simulink model "aircraft_simulation_slc_ff"  (R2016b)
settings: Solver=ode5  StartTime=0.0  StopTime=10000  FixedStep=0.1  RelTol=1e-3  EnableMultiTasking=on
values from neighbouring files (symbols this model uses):
  chi_c = 180/pi*uu(28)    [PlotStateVariables.m]    (also in SLCWithFeedForwardAutopilot.m = uu(19,1); SLCWithFeedForwardAutopilotOLD.m = uu(21,1); SimpleCircleFollow.m = chi_0 + circle_gain_struct.flag*atan(circle_gain_struct.gain; SimpleSLCAutopilot.m = uu(17,1))
  chi_dot_c = uu(18,1)    [SLCWithFeedForwardAutopilot.m]    (also in SLCWithFeedForwardAutopilotOLD.m = control_gain_struct.Kff_course_rate*chi_dot_ff + control_gai; SimpleCircleFollow.m = scale_factor*circle_gain_struct.speed/circle_gain_struct.rad)
  h_c = uu(22)    [PlotStateVariables.m]    (also in SLCWithFeedForwardAutopilot.m = uu(17,1); SLCWithFeedForwardAutopilotOLD.m = uu(19,1); SimpleCircleFollow.m = -circle_gain_struct.center(3,1); SimpleSLCAutopilot.m = uu(18,1))
  h_dot_c = uu(16,1)    [SLCWithFeedForwardAutopilot.m]    (also in SLCWithFeedForwardAutopilotOLD.m = uu(20,1); SimpleCircleFollow.m = 0)
  Va_c = uu(23)    [PlotStateVariables.m]    (also in SLCWithFeedForwardAutopilot.m = uu(20,1); SLCWithFeedForwardAutopilotOLD.m = uu(23,1); SimpleCircleFollow.m = circle_gain_struct.speed; SimpleSLCAutopilot.m = uu(16,1))
  wind_inertial = uu(17:19, 1)    [PlotStateVariables.m]    (also in SLCWithFeedForwardAutopilot.m = uu(13:15,1); S_AircraftForcesAndMoments.m = u(17:19,1); SimpleSLCAutopilot.m = uu(13:15,1))
undefined symbols (not defined in the file or in its folder): aircraft_parameters, circle_gain_struct, control_gain_struct, DRAW_FLAG, drawAircraft, PlotStateVariables, pts, S_AircraftForcesAndMoments, SimpleCircleFollow, SLCWithFeedForwardAutopilot
libraries: aerolibobsolete x1, aerolibatmos2 x1
settings Model: Creator=beard  LastModifiedBy=ericfrew
settings DataIOCC: LimitDataPoints=on  SaveFormat=Array  SignalLoggingSaveFormat=ModelDataLogs
settings OptimizationCC: ExpressionDepthLimit=2147483647  InitFltsAndDblsToZero=on  LifeSpan=inf
settings DebuggingCC: UnderspecifiedInitializationDetection=Classic  MergeDetectMultiDrivingBlocksExec=none  SolverPrmCheckMsg=warning  FcnCallInpInsideContextMsg=warning  StateNameClashWarn=warning  SFUnexpectedBacktrackingDiag=warning  SFNoUnconditionalDefaultTransitionDiag=warning  SFExecutionAtInitializationDiag=none
settings HardwareCC: ProdBitPerPointer=32  ProdBitPerSizeT=32  ProdBitPerPtrDiffT=32  ProdLargestAtomicFloat=None  ProdIntDivRoundTo=Undefined  ProdEndianess=Unspecified  ProdWordSize=32  ProdHWDeviceType=32-bit Generic
settings ModelReferenceCC: PropagateSignalLabelsOutOfModel=off
settings GRTTargetCC: TargetLangStandard=C89/C90 (ANSI)  GeneratePreprocessorConditionals=Disable all  CombineOutputUpdateFcns=off  GRTInterface=on
settings ConfigComp: CovMetricSettings=dw  CovHtmlReporting=on  CovSaveCumulativeToWorkspaceVar=on  CovSaveSingleToWorkspaceVar=on  CovExternalEMLEnable=off  CovSFcnEnable=off

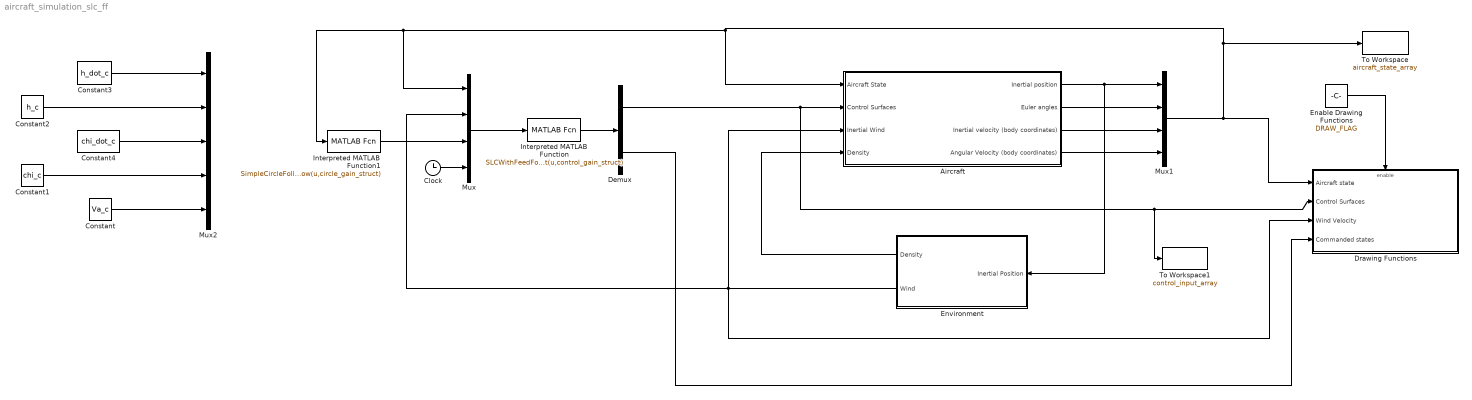
== system aircraft_simulation_slc_ff ==
  Aircraft : Subsystem
  Clock : Clock
  Constant : Constant  Value=Va_c
  Constant1 : Constant  Value=chi_c
  Constant2 : Constant  Value=h_c
  Constant3 : Constant  Value=h_dot_c
  Constant4 : Constant  Value=chi_dot_c
  Demux : Demux  Outputs=[4; 12]
  Drawing Functions : Subsystem  TreatAsAtomicUnit=on
  Enable Drawing Functions : Constant  Value=DRAW_FLAG
  Environment : Subsystem
  Interpreted MATLAB Function : MATLABFcn  MATLABFcn=SLCWithFeedForwardAutopilot(u,control_gain_struct)  OutputDimensions=16  OutputSignalType=real
  Interpreted MATLAB Function1 : MATLABFcn  MATLABFcn=SimpleCircleFollow(u,circle_gain_struct)  OutputDimensions=5  OutputSignalType=real
  Mux : Mux
  Mux1 : Mux
  Mux2 : Mux  Inputs=5
  To Workspace : ToWorkspace  VariableName=aircraft_state_array  SaveFormat=Timeseries  SampleTime=-1
  To Workspace1 : ToWorkspace  VariableName=control_input_array  SaveFormat=Timeseries  SampleTime=-1
  wires:
  Mux1/1 -> Drawing Functions/1(Aircraft state), Interpreted MATLAB Function1/1, Mux/1, Aircraft/1(Aircraft State), To Workspace/1
  Environment/1(Density) -> Aircraft/4(Density)
  Environment/2(Wind) -> Mux/2, Drawing Functions/3(Wind Velocity), Aircraft/3(Inertial Wind)
  Aircraft/4(Angular Velocity (body coordinates)) -> Mux1/4
  Aircraft/3(Inertial velocity (body coordinates)) -> Mux1/3
  Aircraft/2(Euler angles) -> Mux1/2
  Aircraft/1(Inertial position) -> Mux1/1, Environment/1(Inertial Position)
  Demux/1 -> Drawing Functions/2(Control Surfaces), To Workspace1/1, Aircraft/2(Control Surfaces)
  Enable Drawing Functions/1 -> Drawing Functions/Enable
  Demux/2 -> Drawing Functions/4(Commanded states)
  Interpreted MATLAB Function/1 -> Demux/1
  Mux/1 -> Interpreted MATLAB Function/1
  Clock/1 -> Mux/4
  Constant/1 -> Mux2/5
  Constant3/1 -> Mux2/1
  Constant2/1 -> Mux2/2
  Constant1/1 -> Mux2/4
  Constant4/1 -> Mux2/3
  Interpreted MATLAB Function1/1 -> Mux/3

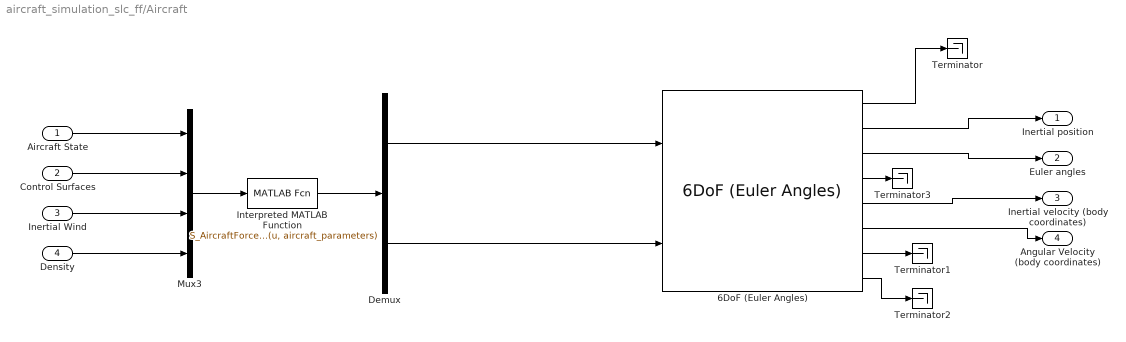
== system aircraft_simulation_slc_ff/Aircraft ==
  Aircraft State : Inport
  Control Surfaces : Inport  Port=2
  Inertial Wind : Inport  Port=3
  Density : Inport  Port=4
  6DoF (Euler Angles) : aerolibobsolete/6DoF (Euler Angles)  units=Metric (MKS)  mtype=Fixed  rep=Euler Angles  xme_0=position_inertial  Vm_0=velocity_body  eul_0=euler_angles  pm_0=omega_body  mass_0=aircraft_parameters.m  mass_e=0.5  mass_f=2.0  inertia=inertia_matrix  inertia_e=eye(3)  inertia_f=2*eye(3)  k_quat=1.0
  Demux : Demux  Outputs=2
  Interpreted MATLAB Function : MATLABFcn  MATLABFcn=S_AircraftForcesAndMoments(u, aircraft_parameters)  OutputDimensions=6
  Mux3 : Mux
  Terminator{,1..3} (4 alike) : Terminator
  Inertial position : Outport
  Euler angles : Outport  Port=2
  Inertial velocity (body coordinates) : Outport  Port=3
  Angular Velocity (body coordinates) : Outport  Port=4
  wires:
  6DoF (Euler Angles)/2 -> Inertial position/1
  6DoF (Euler Angles)/3 -> Euler angles/1
  6DoF (Euler Angles)/5 -> Inertial velocity (body coordinates)/1
  6DoF (Euler Angles)/6 -> Angular Velocity (body coordinates)/1
  Demux/1 -> 6DoF (Euler Angles)/1
  Mux3/1 -> Interpreted MATLAB Function/1
  Demux/2 -> 6DoF (Euler Angles)/2
  Interpreted MATLAB Function/1 -> Demux/1
  Control Surfaces/1 -> Mux3/2
  6DoF (Euler Angles)/1 -> Terminator/1
  6DoF (Euler Angles)/7 -> Terminator1/1
  6DoF (Euler Angles)/8 -> Terminator2/1
  Aircraft State/1 -> Mux3/1
  Inertial Wind/1 -> Mux3/3
  Density/1 -> Mux3/4
  6DoF (Euler Angles)/4 -> Terminator3/1

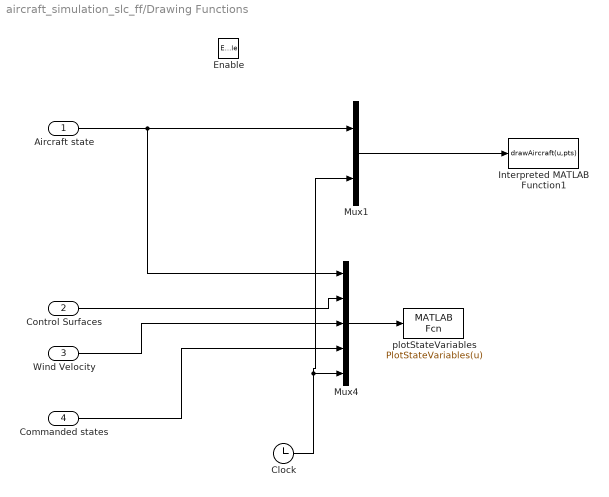
== system aircraft_simulation_slc_ff/Drawing Functions ==
  Aircraft state : Inport
  Control Surfaces : Inport  Port=2
  Wind Velocity : Inport  Port=3
  Commanded states : Inport  Port=4
  Enable : EnablePort
  Clock : Clock
  Interpreted MATLAB Function1 : MATLABFcn  MATLABFcn=drawAircraft(u,pts)  OutputDimensions=0
  Mux1 : Mux  Inputs=2
  Mux4 : Mux  Inputs=5
  plotStateVariables : MATLABFcn  MATLABFcn=PlotStateVariables(u)  OutputDimensions=0
  wires:
  Mux4/1 -> plotStateVariables/1
  Control Surfaces/1 -> Mux4/2
  Wind Velocity/1 -> Mux4/3
  Clock/1 -> Mux1/2, Mux4/5
  Aircraft state/1 -> Mux1/1, Mux4/1
  Mux1/1 -> Interpreted MATLAB Function1/1
  Commanded states/1 -> Mux4/4

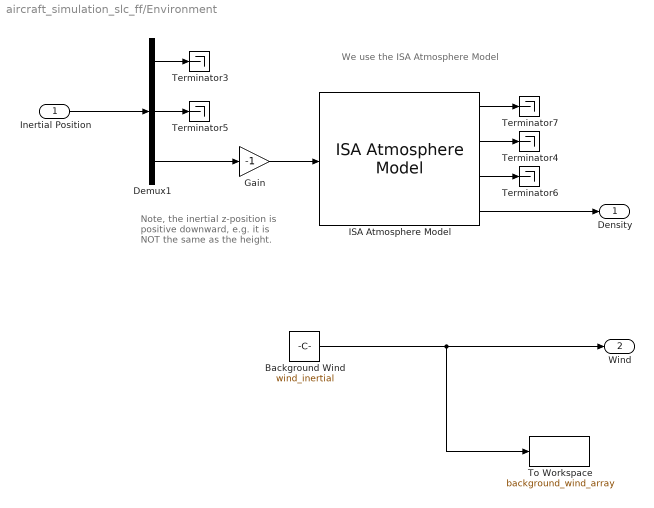
== system aircraft_simulation_slc_ff/Environment ==
  note: Note, the inertial z-position is
      | positive downward, e.g. it is
      | NOT the same as the height.
  note: We use the ISA Atmosphere Model
  Inertial Position : Inport
  Background Wind : Constant  Value=wind_inertial
  Demux1 : Demux  Outputs=3
  Gain : Gain  Gain=-1
  ISA Atmosphere Model : aerolibatmos2/ISA Atmosphere Model  custom=off  g=9.80665  gamma=1.4  R=287.0531  L=0.0065  h_trop=11000  h_strat=20000  rho0=1.225  P0=101325  T0=288.15  h0=0
  Terminator{3..7} (5 alike) : Terminator
  To Workspace : ToWorkspace  VariableName=background_wind_array  SaveFormat=Timeseries  SampleTime=-1
  Density : Outport
  Wind : Outport  Port=2
  wires:
  Inertial Position/1 -> Demux1/1
  Demux1/3 -> Gain/1
  Gain/1 -> ISA Atmosphere Model/1
  Demux1/1 -> Terminator3/1
  Demux1/2 -> Terminator5/1
  ISA Atmosphere Model/3 -> Terminator6/1
  ISA Atmosphere Model/2 -> Terminator4/1
  ISA Atmosphere Model/1 -> Terminator7/1
  ISA Atmosphere Model/4 -> Density/1
  Background Wind/1 -> To Workspace/1, Wind/1
